simulink model "PID_Controller"  (R2024b)
settings: Solver=VariableStepAuto  StartTime=0.0  StopTime=10.0  RelTol=1e-3
undefined symbols (not defined in the file): B, J, k, Kb, Kd, ki, Kp, L, R, Ts
libraries: slpidlib x1
settings Model: Creator=Sagar  LastModifiedBy=Sagar

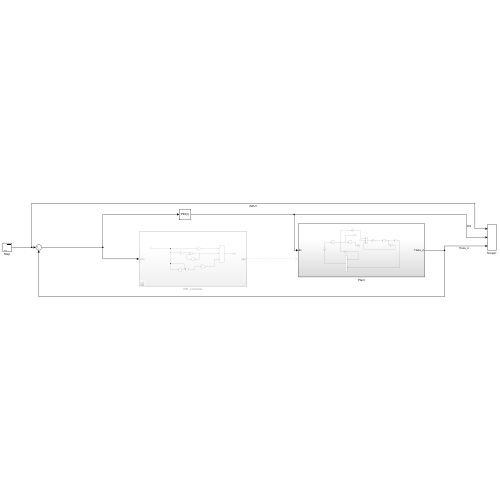
[thumbnail: Simulink's stored preview of the top-level diagram]
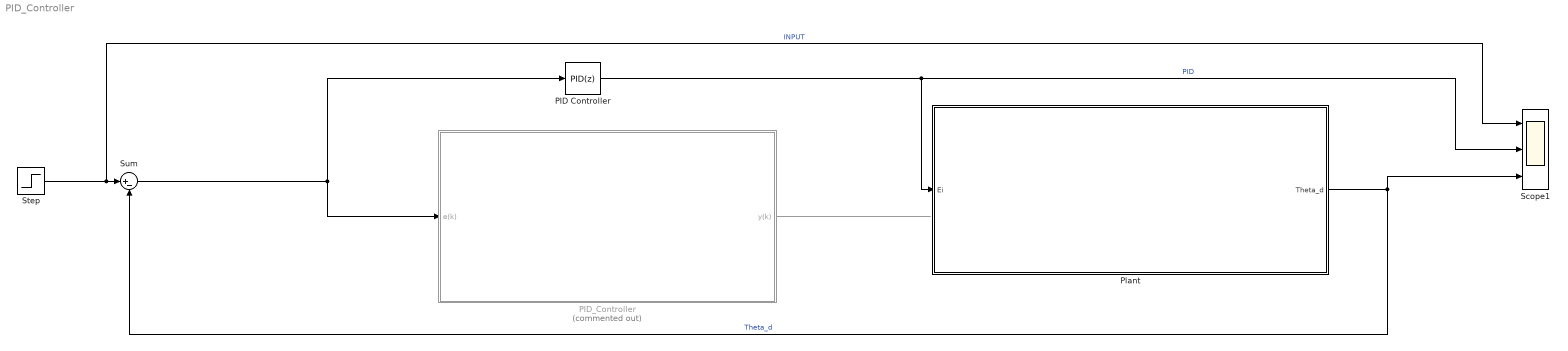
== system PID_Controller ==
  PID Controller : slpidlib/PID Controller  Controller=PID  Form=Parallel  TimeDomain=Discrete-time  UseExternalTs=off  SampleTime=0.01  IntegratorMethod=Forward Euler  FilterMethod=Forward Euler  ControllerParametersSource=internal  P=6.76212612578352  I=19.9942005750745  UseKiTs=off  D=-1.30084947883852  UseExternalDerivativeSource=off  N=4.99351940718644  UseFilter=on  TunerSelectOption=Transfer Function Based (PID Tuner App)  InitialConditionSource=internal  InitialConditionForIntegrator=0  InitialConditionForFilter=0  DifferentiatorICPrevScaledInput=0  ExternalReset=none  TrackingMode=off  Kt=1  LimitOutput=off  SatLimitsSource=internal  UpperSaturationLimit=inf  LowerSaturationLimit=-inf  LinearizeAsGain=on  AntiWindupMode=none  Kb=1  LimitIntegrator=off  UpperIntegratorSaturationLimit=inf  LowerIntegratorSaturationLimit=-inf  POutMin=[]  POutMax=[]  IOutMin=[]  IOutMax=[]  DOutMin=[]  DOutMax=[]  NOutMin=[]  NOutMax=[]  SumOutMin=[]  SumOutMax=[]  SaturationOutMin=[]  SaturationOutMax=[]  PParamMin=[]  PParamMax=[]  IParamMin=[]  IParamMax=[]  DParamMin=[]  DParamMax=[]  NParamMin=[]  NParamMax=[]  KbParamMin=[]  KbParamMax=[]  KtParamMin=[]  KtParamMax=[]  KbOutMin=[]  KbOutMax=[]  KtOutMin=[]  KtOutMax=[]  IntegratorOutMin=[]  IntegratorOutMax=[]  FilterOutMin=[]  FilterOutMax=[]  SumI1OutMin=[]  SumI1OutMax=[]  SumI2OutMin=[]  SumI2OutMax=[]  SumI3OutMin=[]  SumI3OutMax=[]  SumI4OutMin=[]  SumI4OutMax=[]  SumDOutMin=[]  SumDOutMax=[]  DifferentiatorOutMin=[]  DifferentiatorOutMax=[]  FilterDiffOutCoefMin=[]  FilterDiffOutCoefMax=[]  ReciprocalOutMin=[]  ReciprocalOutMax=[]  SumDenOutMin=[]  SumDenOutMax=[]  SumNumOutMin=[]  SumNumOutMax=[]  DivideOutMin=[]  DivideOutMax=[]  UdiffTsProdOutMin=[]  UdiffTsProdOutMax=[]  NTsProdOutMin=[]  NTsProdOutMax=[]  UintegralTsProdOutMin=[]  UintegralTsProdOutMax=[]  UngainTsProdOutMin=[]  UngainTsProdOutMax=[]  ClampingZeroOutDataTypeStr=Inherit: Inherit via back propagation  ClampingZeroOutMin=[]  ClampingZeroOutMax=[]  FilterDenConstantOutDataTypeStr=Inherit: Inherit via back propagation  FilterDenConstantOutMin=[]  FilterDenConstantOutMax=[]  PCopyOutDataTypeStr=Inherit: Inherit via back propagation  PCopyOutMin=[]  PCopyOutMax=[]  NCopyOutDataTypeStr=Inherit: Inherit via back propagation  NCopyOutMin=[]  NCopyOutMax=[]  IntegratorContinuousStateAttributes=''  IntegratorStateMustResolveToSignalObject=off  IntegratorRTWStateStorageClass=Auto  FilterContinuousStateAttributes=''  FilterStateMustResolveToSignalObject=off  FilterRTWStateStorageClass=Auto  ParallelPVariant=InternalParameters  IdealPVariant=Disabled  IVariant=InternalParameters  DVariant=InternalParameters  IntegratorVariant=Discrete  SatVariant=Disabled  AWVariant=Passthrough  PCopyVariant=Disabled  TRVariant=Disabled  FdbkBlocksVariant=Forward  IdealPFdbkVariant=Disabled  SatFdbkVariant=Disabled  DerivativeFilterVariant=ForwardEulerFilter  NVariant=InternalParameters  NCopyVariant=Disabled  FilterICVariant=InternalICsFilter  IntegratorICVariant=InternalICs  ExternalResetVariant=Disabled  TRSumVariant=Passthrough  SumFdbkVariant=Disabled  SumVariant=Sum_PID  TsampFilterVariant=InternalTs  TsampNgainVariant=Passthrough  TsampIntegralVariant=Disabled_SignalSpec  ExternalSaturationOutDataTypeStr=Inherit: Same as second input  DerivativeSourceVariant=ErrorSignal  PreIntVariant=InternalPreInt
  PID_Controller : Subsystem  Commented=on
  Plant : Subsystem
  Scope1 : Scope  NumInputPorts=3
  Step : Step  SampleTime=0
  Sum : Sum  Inputs=|+-
  wires:
  PID Controller/1 -> Plant/1(Ei), Scope1/2  "PID"
  PID_Controller/1(y(k)) -> ?
  Sum/1 -> PID Controller/1, PID_Controller/1(e(k))
  Step/1 -> Scope1/1, Sum/1  "INPUT"
  Plant/1(Theta_d) -> Sum/2, Scope1/3  "Theta_d"

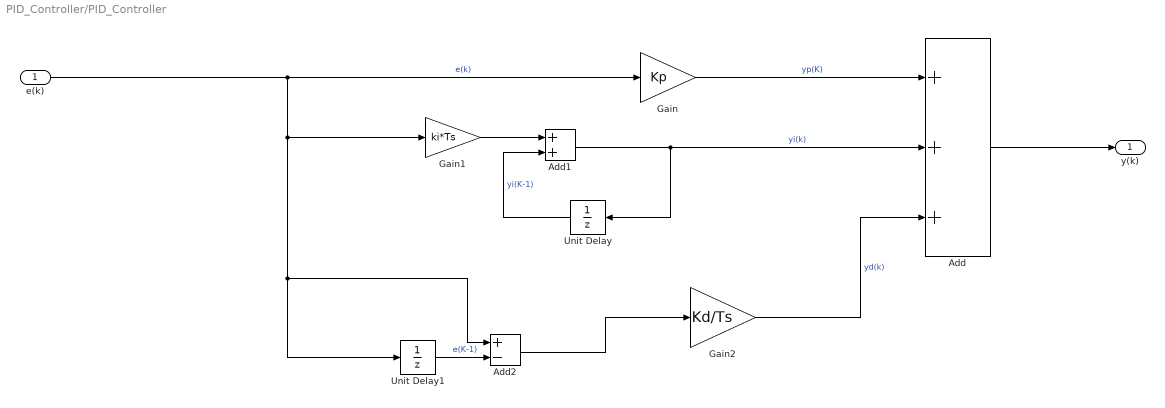
== system PID_Controller/PID_Controller ==
  e(k) : Inport
  Add : Sum  Inputs=+++
  Add1 : Sum
  Add2 : Sum  Inputs=+-
  Gain : Gain  Gain=Kp
  Gain1 : Gain  Gain=ki*Ts
  Gain2 : Gain  Gain=Kd/Ts
  Unit Delay : UnitDelay  SampleTime=-1  HasFrameUpgradeWarning=on
  Unit Delay1 : UnitDelay  SampleTime=-1  HasFrameUpgradeWarning=on
  y(k) : Outport
  wires:
  e(k)/1 -> Add2/1, Unit Delay1/1, Gain1/1, Gain/1  "e(k)"
  Gain/1 -> Add/1  "yp(K)"
  Gain1/1 -> Add1/1
  Add1/1 -> Unit Delay/1, Add/2  "yi(k)"
  Unit Delay/1 -> Add1/2  "yi(K-1)"
  Add/1 -> y(k)/1
  Gain2/1 -> Add/3  "yd(k)"
  Unit Delay1/1 -> Add2/2  "e(K-1)"
  Add2/1 -> Gain2/1

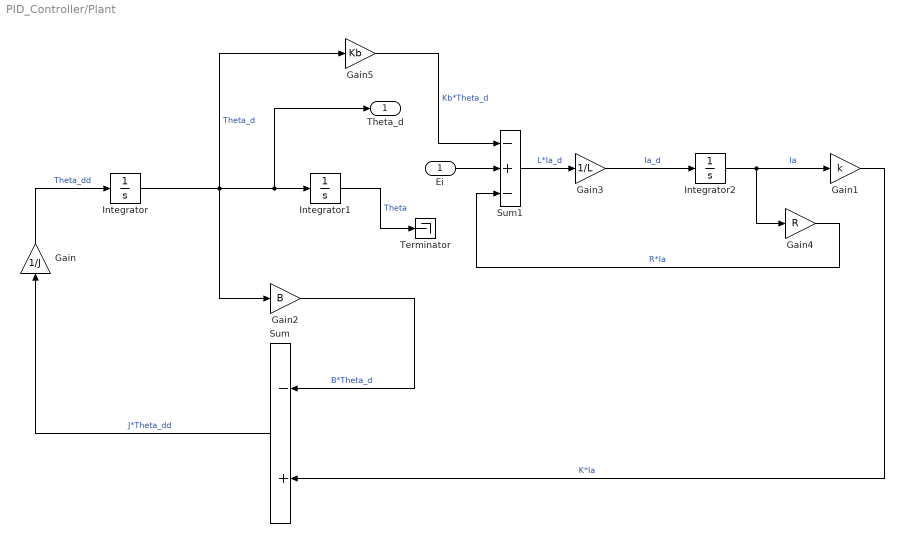
== system PID_Controller/Plant ==
  Ei : Inport
  Gain : Gain  Gain=1/J
  Gain1 : Gain  Gain=k
  Gain2 : Gain  Gain=B
  Gain3 : Gain  Gain=1/L
  Gain4 : Gain  Gain=R
  Gain5 : Gain  Gain=Kb
  Integrator : Integrator
  Integrator1 : Integrator
  Integrator2 : Integrator
  Sum : Sum  Inputs=-+
  Sum1 : Sum  Inputs=-+-
  Terminator : Terminator
  Theta_d : Outport
  wires:
  Integrator/1 -> Gain2/1, Theta_d/1, Integrator1/1, Gain5/1  "Theta_d"
  Sum/1 -> Gain/1  "J*Theta_dd"
  Integrator2/1 -> Gain1/1, Gain4/1  "Ia"
  Gain1/1 -> Sum/2  "K*Ia"
  Gain3/1 -> Integrator2/1  "Ia_d"
  Gain/1 -> Integrator/1  "Theta_dd"
  Sum1/1 -> Gain3/1  "L*Ia_d"
  Ei/1 -> Sum1/2
  Gain5/1 -> Sum1/1  "Kb*Theta_d"
  Gain4/1 -> Sum1/3  "R*Ia"
  Gain2/1 -> Sum/1  "B*Theta_d"
  Integrator1/1 -> Terminator/1  "Theta"
